simulink library "xblocks_library_ffts_internal"  (Simulink 7.4)
settings: Solver=ode45  StartTime=0.0  StopTime=10.0  RelTol=1e-3
libraries: xbsIndex_r4 x535
(part 1 of 5)
settings Model: Creator=wjm  LastModifiedBy=chenhong

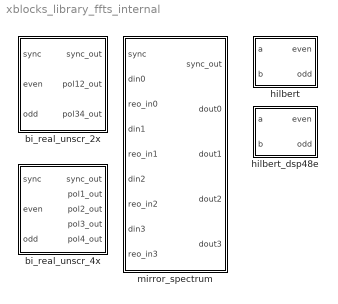
== system xblocks_library_ffts_internal ==
  bi_real_unscr_2x : Subsystem  mask(bi_real_unscr_2x){FFTSize=2, n_bits=18, add_latency=1, conv_latency=1, bram_latency=2, bram_map=off, dsp48_adders=off}
      mask prompts: FFTSize "Size of FFT (2^?):"; n_bits "Sample Bit Width"; add_latency "Add Latency"; conv_latency "Convert Latency"; bram_latency "BRAM Latency"; bram_map "Use BlockRAM for Map"; dsp48_adders "Use DSP48s for adders"
      mask help:
      | FFT internal block.
      |
      | (xBlock version)
      mask init:
      | config.source = str2func('fft_bi_real_unscr_2x_init_xblock');
      | config.toplevel = gcb;
      | config.depend = get_dependlist('fft_bi_real_unscr_2x');
      | set_param(gcb,'LinkStatus','inactive');
      | xBlock( config, {config.toplevel,...
      |     'FFTSize', FFTSize, ...
      |     'n_bits', n_bits, ...
      |     'add_latency', add_latency, ...
      |     'conv_latency', conv_latency, ...
      |     'bram_latency', bram_latency, ...
      |     'bram_map', bram_map, ...
      |     'dsp48_adders', dsp48_adders});
      settings: AttributesFormatString=18_17 r/i
      mask TabNameString: Basic,Basic,Latency,Latency,Latency,Implementation,Implementation
  bi_real_unscr_4x : Subsystem  mask(bi_real_unscr_4x){FFTSize=8, n_bits=18, add_latency=1, conv_latency=1, bram_latency=2, bram_map=off, bram_delays=off, dsp48_adders=on}
      mask prompts: FFTSize "Size of FFT (2^?):"; n_bits "Sample Bit Width"; add_latency "Add Latency"; conv_latency "Convert Latency"; bram_latency "BRAM Latency"; bram_map "Use BlockRAM for Map"; bram_delays "Use BlockRAM for Delays"; dsp48_adders "Use DSP48s for adders"
      mask help:
      | FFT internal block.
      |
      | (xBlock version)
      mask init:
      | config.source = str2func('fft_bi_real_unscr_4x_init_xblock');
      | config.toplevel = gcb;
      | config.depend = get_dependlist('fft_bi_real_unscr_4x');
      | set_param(gcb,'LinkStatus','inactive');
      | xBlock( config, {config.toplevel,...
      |     'FFTSize', FFTSize, ...
      |     'n_bits', n_bits, ...
      |     'add_latency', add_latency, ...
      |     'conv_latency', conv_latency, ...
      |     'bram_latency', bram_latency, ...
      |     'bram_map', bram_map, ...
      |     'bram_delays', bram_delays, ...
      |     'dsp48_adders', dsp48_adders});
      mask TabNameString: Basic,Basic,Latency,Latency,Latency,Implementation,Implementation,Implementation
  hilbert : Subsystem  mask(hilbert (xBlock)){BitWidth=16, add_latency=2, conv_latency=2}
      mask prompts: BitWidth "Bit Wdith"; add_latency "Add Latency"; conv_latency "Convert Latency"
      mask help:
      | FFT internal block.
      |
      | Computes (a+b*)/2 and (a-b*)/2i.
      |
      | If a = w + ix and b = y + iz, then:
      | a+b = (w+y)/2 + i(x-z)/2
      | a-b = (x+z)/2 + i(y-w)/2
      mask init:
      | config.source = str2func('hilbert_init_xblock');
      | config.toplevel = gcb;
      | config.depend = get_dependlist('hilbert');
      | set_param(gcb,'LinkStatus','inactive');
      | xBlock( config, {config.toplevel, ...
      |     BitWidth, add_latency, conv_latency});
  hilbert_dsp48e : Subsystem  mask(sincos_dsp48e (xBlock version)){BitWidth=16, conv_latency=2}
      mask prompts: BitWidth "Bit Wdith"; conv_latency "Convert Latency"
      mask help:
      | FFT internal block.
      |
      | Computes (a+b*)/2 and (a-b*)/2i.
      mask init:
      | config.source = str2func('hilbert_dsp48e_init_xblock');
      | config.toplevel = gcb;
      | config.depend = get_dependlist('hilbert_dsp48e');
      | set_param(gcb,'LinkStatus','inactive');
      | xBlock(config, {config.toplevel, ...
      |     BitWidth, conv_latency});
  mirror_spectrum : Subsystem  mask(mirror_spectrum){FFTSize=8, input_bitwidth=18, bram_latency=2, negate_latency=1, negate_mode=logic}
      mask prompts: FFTSize "Size of FFT (2^?)"; input_bitwidth "Input Bit Width"; bram_latency "BRAM Latency"; negate_latency "Negate Latency"; negate_mode "Negate mode"
      mask help: FFT internal block.
      mask init:
      | config.source = str2func('mirror_spectrum_init_xblock');
      | config.toplevel = gcb;
      | config.depend = get_dependlist('mirror_spectrum');
      | set_param(gcb,'LinkStatus','inactive');
      | xBlock( config, {config.toplevel, ...
      |     FFTSize, input_bitwidth,...
      |     bram_latency, negate_latency, ...
      |     negate_mode});
      settings: AttributesFormatString=18_17 r/i
      mask StyleString: edit,edit,edit,edit,popup(dsp48e|logic)
      mask TabNameString: Basic,Basic,Latency,Latency,Latency

== system xblocks_library_ffts_internal/bi_real_unscr_2x ==
  sync : Inport  OutDataType=sfix(16)  OutScaling=2^0
  even : Inport  Port=2  OutDataType=sfix(16)  OutScaling=2^0
  odd : Inport  Port=3  OutDataType=sfix(16)  OutScaling=2^0
  Constant : xbsIndex_r4/Constant  arith_type=Unsigned  const=0  n_bits=1  bin_pt=0  explicit_period=on  period=1  equ=P=C  opselect=C  inp2=PCIN>>17  opr=+  inp1=P  carry=CIN  dbl_ovrd=off  block_type=constant
      settings: block_version=11.4
  Counter : xbsIndex_r4/Counter  cnt_type=Free Running  cnt_to=Inf  operation=Up  start_count=0  cnt_by_val=1  arith_type=Unsigned  n_bits=1  bin_pt=0  load_pin=off  rst=on  en=off  explicit_period=on  period=1  dbl_ovrd=off  use_behavioral_HDL=off  implementation=Fabric  block_type=counter
      settings: block_version=11.4
  Delay : xbsIndex_r4/Delay  en=off  latency=1  dbl_ovrd=off  reg_retiming=off  block_type=delay
      settings: block_version=11.4
  Mux : xbsIndex_r4/Mux  inputs=2  en=off  latency=0  precision=Full  arith_type="Signed  (2's comp)"  n_bits=8  bin_pt=2  quantization=Truncate  overflow=Wrap  dbl_ovrd=off  block_type=mux
      settings: block_version=11.4
  Relational : xbsIndex_r4/Relational  mode=a=b  en=off  latency=0  dbl_ovrd=off  block_type=relational
  en_even : xbsIndex_r4/Constant  arith_type=Boolean  const=1  n_bits=1  bin_pt=0  explicit_period=on  period=1  equ=P=C  opselect=C  inp2=PCIN>>17  opr=+  inp1=P  carry=CIN  dbl_ovrd=off  block_type=constant
      settings: block_version=11.4
  en_odd : xbsIndex_r4/Constant  arith_type=Boolean  const=1  n_bits=1  bin_pt=0  explicit_period=on  period=1  equ=P=C  opselect=C  inp2=PCIN>>17  opr=+  inp1=P  carry=CIN  dbl_ovrd=off  block_type=constant
      settings: block_version=11.4
  hilbert : Subsystem
      settings: AttributesFormatString=18_17 r/i
  reorder_even : Subsystem
      settings: AttributesFormatString=order=1
  reorder_odd : Subsystem
      settings: AttributesFormatString=order=2
  sync_delay : xbsIndex_r4/Delay  en=off  latency=2  dbl_ovrd=off  reg_retiming=off  block_type=delay
      settings: block_version=11.4
  sync_out : Outport  OutDataType=sfix(16)  OutScaling=2^0
  pol12_out : Outport  Port=2  OutDataType=sfix(16)  OutScaling=2^0
  pol34_out : Outport  Port=3  OutDataType=sfix(16)  OutScaling=2^0
  wires:
  sync/1 -> reorder_odd/1(sync), reorder_even/1(sync)
  reorder_even/1(sync_out) -> sync_delay/1, Counter/1
  reorder_even/3(dout0) -> hilbert/1(a), Mux/3
  reorder_odd/3(dout0) -> Delay/1
  odd/1 -> reorder_odd/3(din0)
  en_odd/1 -> reorder_odd/2(en)
  even/1 -> reorder_even/3(din0)
  en_even/1 -> reorder_even/2(en)
  hilbert/2(odd) -> pol34_out/1
  hilbert/1(even) -> pol12_out/1
  Mux/1 -> hilbert/2(b)
  sync_delay/1 -> sync_out/1
  Relational/1 -> Mux/1
  Constant/1 -> Relational/2
  Counter/1 -> Relational/1
  Delay/1 -> Mux/2

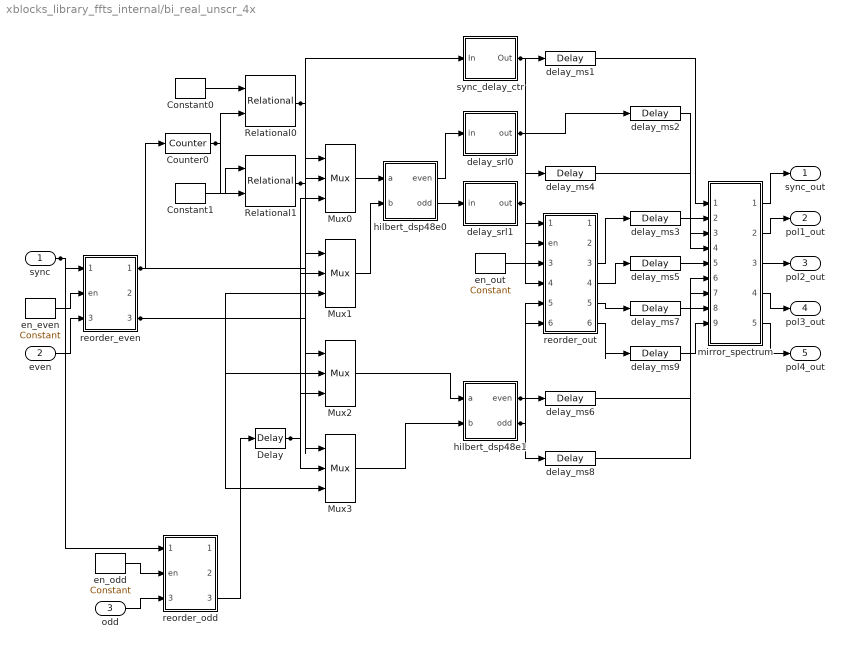
== system xblocks_library_ffts_internal/bi_real_unscr_4x ==
  sync : Inport
  even : Inport  Port=2
  odd : Inport  Port=3
  Constant0 : xbsIndex_r4/Constant  arith_type=Unsigned  const=128  n_bits=8  bin_pt=0  explicit_period=on  period=1  equ=P=C  opselect=C  inp2=PCIN>>17  opr=+  inp1=P  carry=CIN  dbl_ovrd=off  block_type=constant
      settings: block_version=11.4
  Constant1 : xbsIndex_r4/Constant  arith_type=Unsigned  const=0  n_bits=8  bin_pt=0  explicit_period=on  period=1  equ=P=C  opselect=C  inp2=PCIN>>17  opr=+  inp1=P  carry=CIN  dbl_ovrd=off  block_type=constant
      settings: block_version=11.4
  Counter0 : xbsIndex_r4/Counter  cnt_type=Free Running  cnt_to=Inf  operation=Up  start_count=0  cnt_by_val=1  arith_type=Unsigned  n_bits=8  bin_pt=0  load_pin=off  rst=on  en=off  explicit_period=on  period=1  dbl_ovrd=off  use_behavioral_HDL=off  implementation=Fabric  block_type=counter
      settings: block_version=11.4
  Delay : xbsIndex_r4/Delay  en=off  latency=1  dbl_ovrd=off  reg_retiming=off  block_type=delay
      settings: block_version=11.4
  Mux{0..3} (4 alike) : xbsIndex_r4/Mux  inputs=2  en=off  latency=1  precision=Full  arith_type=Unsigned  n_bits=16  bin_pt=14  quantization=Truncate  overflow=Wrap  dbl_ovrd=off  block_type=mux
      settings: block_version=11.4
  Relational0 : xbsIndex_r4/Relational  mode=a=b  en=off  latency=0  dbl_ovrd=off  block_type=relational
  Relational1 : xbsIndex_r4/Relational  mode=a=b  en=off  latency=0  dbl_ovrd=off  block_type=relational
  delay_ms{1..9} (9 alike) : xbsIndex_r4/Delay  en=off  latency=1  dbl_ovrd=off  reg_retiming=off  block_type=delay
      settings: block_version=11.4
  delay_srl0 : Subsystem
  delay_srl1 : Subsystem
  en_even : xbsIndex_r4/Constant  arith_type=Boolean  const=1  n_bits=1  bin_pt=0  explicit_period=on  period=1  equ=P=C  opselect=C  inp2=PCIN>>17  opr=+  inp1=P  carry=CIN  dbl_ovrd=off  block_type=constant
      settings: block_version=11.4
  en_odd : xbsIndex_r4/Constant  arith_type=Boolean  const=1  n_bits=1  bin_pt=0  explicit_period=on  period=1  equ=P=C  opselect=C  inp2=PCIN>>17  opr=+  inp1=P  carry=CIN  dbl_ovrd=off  block_type=constant
      settings: block_version=11.4
  en_out : xbsIndex_r4/Constant  arith_type=Boolean  const=1  n_bits=1  bin_pt=0  explicit_period=on  period=1  equ=P=C  opselect=C  inp2=PCIN>>17  opr=+  inp1=P  carry=CIN  dbl_ovrd=off  block_type=constant
      settings: block_version=11.4
  hilbert_dsp48e0 : Subsystem
  hilbert_dsp48e1 : Subsystem
  mirror_spectrum : Subsystem
  reorder_even : Subsystem
      settings: AttributesFormatString=order=2
  reorder_odd : Subsystem
      settings: AttributesFormatString=order=2
  reorder_out : Subsystem
      settings: AttributesFormatString=order=2
  sync_delay_ctr : Subsystem
  sync_out : Outport
  pol1_out : Outport  Port=2
  pol2_out : Outport  Port=3
  pol3_out : Outport  Port=4
  pol4_out : Outport  Port=5
  wires:
  sync/1 -> reorder_odd/1(sync), reorder_even/1(sync)
  reorder_even/1(sync_out) -> sync_delay_ctr/1(In), Counter0/1
  Counter0/1 -> Relational1/2, Relational0/2
  Relational0/1 -> Mux3/1, Mux0/1
  reorder_even/3(dout0) -> Mux3/3, Mux2/2, Mux1/3, Mux0/2
  Delay/1 -> Mux3/2, Mux2/3, Mux1/2, Mux0/3
  Relational1/1 -> Mux2/1, Mux1/1
  sync_delay_ctr/1(Out) -> delay_ms1/1, reorder_out/1(sync)
  delay_srl0/1(out) -> delay_ms2/1, reorder_out/3(din0)
  delay_srl1/1(out) -> delay_ms4/1, reorder_out/4(din1)
  hilbert_dsp48e1/1(even) -> delay_ms6/1, reorder_out/5(din2)
  hilbert_dsp48e1/2(odd) -> delay_ms8/1, reorder_out/6(din3)
  mirror_spectrum/5(dout3) -> pol4_out/1
  mirror_spectrum/4(dout2) -> pol3_out/1
  mirror_spectrum/3(dout1) -> pol2_out/1
  mirror_spectrum/2(dout0) -> pol1_out/1
  mirror_spectrum/1(sync_out) -> sync_out/1
  delay_ms9/1 -> mirror_spectrum/9(reo_in3)
  delay_ms8/1 -> mirror_spectrum/8(din3)
  delay_ms7/1 -> mirror_spectrum/7(reo_in2)
  delay_ms6/1 -> mirror_spectrum/6(din2)
  delay_ms5/1 -> mirror_spectrum/5(reo_in1)
  delay_ms4/1 -> mirror_spectrum/4(din1)
  delay_ms3/1 -> mirror_spectrum/3(reo_in0)
  delay_ms2/1 -> mirror_spectrum/2(din0)
  delay_ms1/1 -> mirror_spectrum/1(sync)
  reorder_out/6(dout3) -> delay_ms9/1
  reorder_out/5(dout2) -> delay_ms7/1
  reorder_out/4(dout1) -> delay_ms5/1
  reorder_out/3(dout0) -> delay_ms3/1
  en_out/1 -> reorder_out/2(en)
  hilbert_dsp48e0/2(odd) -> delay_srl1/1(in)
  hilbert_dsp48e0/1(even) -> delay_srl0/1(in)
  Mux3/1 -> hilbert_dsp48e1/2(b)
  Mux2/1 -> hilbert_dsp48e1/1(a)
  Mux1/1 -> hilbert_dsp48e0/2(b)
  Mux0/1 -> hilbert_dsp48e0/1(a)
  reorder_odd/3(dout0) -> Delay/1
  Constant1/1 -> Relational1/1
  Constant0/1 -> Relational0/1
  odd/1 -> reorder_odd/3(din0)
  en_odd/1 -> reorder_odd/2(en)
  even/1 -> reorder_even/3(din0)
  en_even/1 -> reorder_even/2(en)

== system xblocks_library_ffts_internal/hilbert ==
  a : Inport  OutDataType=sfix(16)  OutScaling=2^0
  b : Inport  Port=2  OutDataType=sfix(16)  OutScaling=2^0
  AddSub : xbsIndex_r4/AddSub  mode=Addition  use_carryin=off  use_carryout=off  en=off  latency=2  precision=Full  arith_type=Unsigned  n_bits=8  bin_pt=2  quantization=Truncate  overflow=Wrap  dbl_ovrd=off  use_behavioral_HDL=on  hw_selection=Fabric  pipelined=off  use_rpm=on  block_type=addsub
  AddSub1 : xbsIndex_r4/AddSub  mode=Subtraction  use_carryin=off  use_carryout=off  en=off  latency=2  precision=Full  arith_type=Unsigned  n_bits=8  bin_pt=2  quantization=Truncate  overflow=Wrap  dbl_ovrd=off  use_behavioral_HDL=on  hw_selection=Fabric  pipelined=off  use_rpm=on  block_type=addsub
  AddSub2 : xbsIndex_r4/AddSub  mode=Subtraction  use_carryin=off  use_carryout=off  en=off  latency=2  precision=Full  arith_type=Unsigned  n_bits=8  bin_pt=2  quantization=Truncate  overflow=Wrap  dbl_ovrd=off  use_behavioral_HDL=on  hw_selection=Fabric  pipelined=off  use_rpm=on  block_type=addsub
  AddSub3 : xbsIndex_r4/AddSub  mode=Addition  use_carryin=off  use_carryout=off  en=off  latency=2  precision=Full  arith_type=Unsigned  n_bits=8  bin_pt=2  quantization=Truncate  overflow=Wrap  dbl_ovrd=off  use_behavioral_HDL=on  hw_selection=Fabric  pipelined=off  use_rpm=on  block_type=addsub
  Convert{,1..3} (4 alike) : xbsIndex_r4/Convert  arith_type="Signed  (2's comp)"  n_bits=16  bin_pt=15  quantization="Round  (unbiased: Even Values)"  overflow=Wrap  latency=2  dbl_ovrd=off  pipeline=off  block_type=convert
      settings: block_version=11.4
  Scale{,1..3} (4 alike) : xbsIndex_r4/Scale  scale_factor=-1  dbl_ovrd=off  block_type=scale
  c_to_ri : Subsystem
      settings: AttributesFormatString=16_15 r/i
  c_to_ri1 : Subsystem
      settings: AttributesFormatString=16_15 r/i
  ri_to_c : Subsystem
  ri_to_c1 : Subsystem
  even : Outport  OutDataType=sfix(16)  OutScaling=2^0
  odd : Outport  Port=2  OutDataType=sfix(16)  OutScaling=2^0
  wires:
  c_to_ri/1(re) -> AddSub1/2, AddSub/1
  c_to_ri/2(im) -> AddSub3/1, AddSub2/1
  c_to_ri1/1(re) -> AddSub1/1, AddSub/2
  c_to_ri1/2(im) -> AddSub3/2, AddSub2/2
  ri_to_c1/1(c) -> odd/1
  Convert1/1 -> ri_to_c1/2(im)
  Convert3/1 -> ri_to_c1/1(re)
  ri_to_c/1(c) -> even/1
  Convert2/1 -> ri_to_c/2(im)
  Convert/1 -> ri_to_c/1(re)
  b/1 -> c_to_ri1/1(c)
  a/1 -> c_to_ri/1(c)
  Scale3/1 -> Convert3/1
  AddSub3/1 -> Scale3/1
  Scale2/1 -> Convert2/1
  AddSub2/1 -> Scale2/1
  Scale1/1 -> Convert1/1
  AddSub1/1 -> Scale1/1
  Scale/1 -> Convert/1
  AddSub/1 -> Scale/1

== system xblocks_library_ffts_internal/hilbert_dsp48e ==
  a : Inport
  b : Inport  Port=2
  Convert{0..3} (4 alike) : xbsIndex_r4/Convert  arith_type="Signed  (2's comp)"  n_bits=16  bin_pt=15  quantization="Round  (unbiased: Even Values)"  overflow=Wrap  latency=2  dbl_ovrd=off  pipeline=on  block_type=convert
      settings: block_version=11.4
  Scale{0..3} (4 alike) : xbsIndex_r4/Scale  scale_factor=-1  dbl_ovrd=off  block_type=scale
  c_to_ri0 : Subsystem
      settings: AttributesFormatString=16_15 r/i
  c_to_ri1 : Subsystem
      settings: AttributesFormatString=16_15 r/i
  cadd : Subsystem
      settings: AttributesFormatString=|
      | 16_15 + 16_15 ==> 17_15
      | Mode=Addition
      | Latency=2
  csub : Subsystem
      settings: AttributesFormatString=|
      | 16_15 + 16_15 ==> 17_15
      | Mode=Subtraction
      | Latency=2
  ri_to_c0 : Subsystem
  ri_to_c1 : Subsystem
  even : Outport
  odd : Outport  Port=2
  wires:
  c_to_ri0/1(re) -> csub/4(b_im), cadd/1(a_re)
  c_to_ri0/2(im) -> csub/1(a_re), cadd/2(a_im)
  c_to_ri1/1(re) -> csub/2(a_im), cadd/3(b_re)
  c_to_ri1/2(im) -> csub/3(b_re), cadd/4(b_im)
  ri_to_c1/1(c) -> odd/1
  Convert3/1 -> ri_to_c1/2(im)
  Convert1/1 -> ri_to_c1/1(re)
  ri_to_c0/1(c) -> even/1
  Convert2/1 -> ri_to_c0/2(im)
  Convert0/1 -> ri_to_c0/1(re)
  csub/2(c_im) -> Scale3/1
  csub/1(c_re) -> Scale2/1
  cadd/2(c_im) -> Scale1/1
  cadd/1(c_re) -> Scale0/1
  b/1 -> c_to_ri1/1(c)
  a/1 -> c_to_ri0/1(c)
  Scale3/1 -> Convert3/1
  Scale2/1 -> Convert2/1
  Scale1/1 -> Convert1/1
  Scale0/1 -> Convert0/1

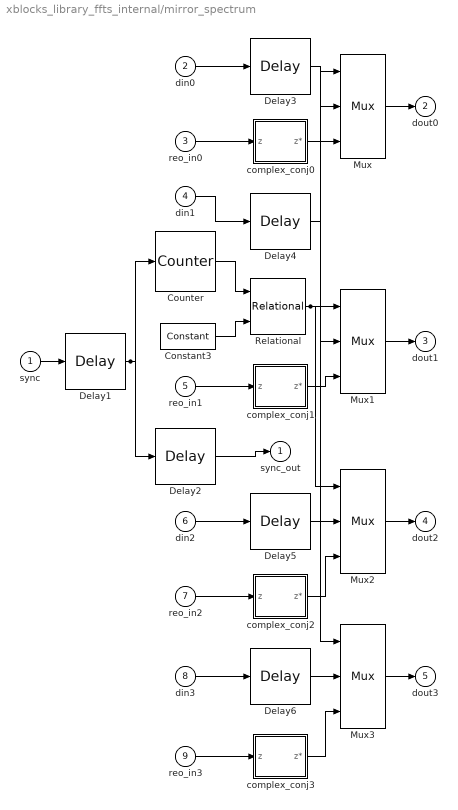
== system xblocks_library_ffts_internal/mirror_spectrum ==
  sync : Inport
  din0 : Inport  Port=2
  reo_in0 : Inport  Port=3
  din1 : Inport  Port=4
  reo_in1 : Inport  Port=5
  din2 : Inport  Port=6
  reo_in2 : Inport  Port=7
  din3 : Inport  Port=8
  reo_in3 : Inport  Port=9
  Constant3 : xbsIndex_r4/Constant  arith_type=Unsigned  const=128  n_bits=8  bin_pt=0  explicit_period=on  period=1  equ=P=C  opselect=C  inp2=PCIN>>17  opr=+  inp1=P  carry=CIN  dbl_ovrd=off  block_type=constant
      settings: block_version=11.4
  Counter : xbsIndex_r4/Counter  cnt_type=Free Running  cnt_to=Inf  operation=Up  start_count=0  cnt_by_val=1  arith_type=Unsigned  n_bits=8  bin_pt=0  load_pin=off  rst=on  en=off  explicit_period=off  period=1  dbl_ovrd=off  use_behavioral_HDL=off  implementation=Fabric  use_rpm=on  block_type=counter
      settings: block_version=11.4
  Delay1 : xbsIndex_r4/Delay  en=off  latency=2  dbl_ovrd=off  reg_retiming=off  block_type=delay
      settings: block_version=11.4
  Delay2 : xbsIndex_r4/Delay  en=off  latency=2  dbl_ovrd=off  reg_retiming=off  block_type=delay
      settings: block_version=11.4
  Delay{3..6} (4 alike) : xbsIndex_r4/Delay  en=off  latency=3  dbl_ovrd=off  reg_retiming=off  block_type=delay
      settings: block_version=11.4
  Mux{,1..3} (4 alike) : xbsIndex_r4/Mux  inputs=2  en=off  latency=1  precision=Full  arith_type="Signed  (2's comp)"  n_bits=8  bin_pt=2  quantization=Truncate  overflow=Wrap  dbl_ovrd=off  block_type=mux
      settings: block_version=11.4
  Relational : xbsIndex_r4/Relational  mode=a>b  en=off  latency=1  dbl_ovrd=off  block_type=relational
  complex_conj0 : Subsystem
      settings: AttributesFormatString=18_17 r/i
  complex_conj1 : Subsystem
      settings: AttributesFormatString=18_17 r/i
  complex_conj2 : Subsystem
      settings: AttributesFormatString=18_17 r/i
  complex_conj3 : Subsystem
      settings: AttributesFormatString=18_17 r/i
  sync_out : Outport
  dout0 : Outport  Port=2
  dout1 : Outport  Port=3
  dout2 : Outport  Port=4
  dout3 : Outport  Port=5
  wires:
  Delay1/1 -> Delay2/1, Counter/1
  Relational/1 -> Mux3/1, Mux2/1, Mux1/1, Mux/1
  complex_conj3/1(z*) -> Mux3/3
  reo_in3/1 -> complex_conj3/1(z)
  complex_conj2/1(z*) -> Mux2/3
  reo_in2/1 -> complex_conj2/1(z)
  complex_conj1/1(z*) -> Mux1/3
  reo_in1/1 -> complex_conj1/1(z)
  complex_conj0/1(z*) -> Mux/3
  reo_in0/1 -> complex_conj0/1(z)
  Constant3/1 -> Relational/2
  Counter/1 -> Relational/1
  Mux3/1 -> dout3/1
  Delay6/1 -> Mux3/2
  Mux2/1 -> dout2/1
  Delay5/1 -> Mux2/2
  Mux1/1 -> dout1/1
  Delay4/1 -> Mux1/2
  Mux/1 -> dout0/1
  Delay3/1 -> Mux/2
  din3/1 -> Delay6/1
  din2/1 -> Delay5/1
  din1/1 -> Delay4/1
  din0/1 -> Delay3/1
  Delay2/1 -> sync_out/1
  sync/1 -> Delay1/1

== system xblocks_library_ffts_internal/bi_real_unscr_2x/hilbert ==
  a : Inport
  b : Inport  Port=2
  AddSub : xbsIndex_r4/AddSub  mode=Addition  use_carryin=off  use_carryout=off  en=off  latency=1  precision=Full  arith_type=Unsigned  n_bits=8  bin_pt=2  quantization=Truncate  overflow=Wrap  dbl_ovrd=off  use_behavioral_HDL=on  hw_selection=Fabric  pipelined=off  use_rpm=on  block_type=addsub
  AddSub1 : xbsIndex_r4/AddSub  mode=Subtraction  use_carryin=off  use_carryout=off  en=off  latency=1  precision=Full  arith_type=Unsigned  n_bits=8  bin_pt=2  quantization=Truncate  overflow=Wrap  dbl_ovrd=off  use_behavioral_HDL=on  hw_selection=Fabric  pipelined=off  use_rpm=on  block_type=addsub
  AddSub2 : xbsIndex_r4/AddSub  mode=Subtraction  use_carryin=off  use_carryout=off  en=off  latency=1  precision=Full  arith_type=Unsigned  n_bits=8  bin_pt=2  quantization=Truncate  overflow=Wrap  dbl_ovrd=off  use_behavioral_HDL=on  hw_selection=Fabric  pipelined=off  use_rpm=on  block_type=addsub
  AddSub3 : xbsIndex_r4/AddSub  mode=Addition  use_carryin=off  use_carryout=off  en=off  latency=1  precision=Full  arith_type=Unsigned  n_bits=8  bin_pt=2  quantization=Truncate  overflow=Wrap  dbl_ovrd=off  use_behavioral_HDL=on  hw_selection=Fabric  pipelined=off  use_rpm=on  block_type=addsub
  Convert{,1..3} (4 alike) : xbsIndex_r4/Convert  arith_type="Signed  (2's comp)"  n_bits=18  bin_pt=17  quantization="Round  (unbiased: Even Values)"  overflow=Wrap  latency=1  dbl_ovrd=off  pipeline=off  block_type=convert
      settings: block_version=11.4
  Scale{,1..3} (4 alike) : xbsIndex_r4/Scale  scale_factor=-1  dbl_ovrd=off  block_type=scale
  c_to_ri : Subsystem
  c_to_ri1 : Subsystem
  ri_to_c : Subsystem
  ri_to_c1 : Subsystem
  even : Outport
  odd : Outport  Port=2
  wires:
  c_to_ri/1(re) -> AddSub1/2, AddSub/1
  c_to_ri/2(im) -> AddSub3/1, AddSub2/1
  c_to_ri1/1(re) -> AddSub1/1, AddSub/2
  c_to_ri1/2(im) -> AddSub3/2, AddSub2/2
  ri_to_c1/1(c) -> odd/1
  Convert1/1 -> ri_to_c1/2(im)
  Convert3/1 -> ri_to_c1/1(re)
  ri_to_c/1(c) -> even/1
  Convert2/1 -> ri_to_c/2(im)
  Convert/1 -> ri_to_c/1(re)
  b/1 -> c_to_ri1/1(c)
  a/1 -> c_to_ri/1(c)
  Scale3/1 -> Convert3/1
  AddSub3/1 -> Scale3/1
  Scale2/1 -> Convert2/1
  AddSub2/1 -> Scale2/1
  Scale1/1 -> Convert1/1
  AddSub1/1 -> Scale1/1
  Scale/1 -> Convert/1
  AddSub/1 -> Scale/1

== system xblocks_library_ffts_internal/bi_real_unscr_2x/reorder_even ==
  sync : Inport
  en : Inport  Port=2
  din0 : Inport  Port=3
  delay_din1 : xbsIndex_r4/Delay  en=off  latency=1  dbl_ovrd=off  reg_retiming=off  block_type=delay
      settings: block_version=11.4
  delay_din_bram0 : Subsystem
  delay_valid : xbsIndex_r4/Delay  en=off  latency=3  dbl_ovrd=off  reg_retiming=off  block_type=delay
      settings: block_version=11.4
  delay_we : xbsIndex_r4/Delay  en=off  latency=0  dbl_ovrd=off  reg_retiming=off  block_type=delay
      settings: block_version=11.4
  post_sync_delay : xbsIndex_r4/Delay  en=off  latency=3  dbl_ovrd=off  reg_retiming=off  block_type=delay
      settings: block_version=11.4
  pre_sync_delay : xbsIndex_r4/Delay  en=off  latency=0  dbl_ovrd=off  reg_retiming=off  block_type=delay
      settings: block_version=11.4
  sync_delay_en : Subsystem
  sync_out : Outport
  valid : Outport  Port=2
  dout0 : Outport  Port=3
  wires:
  en/1 -> delay_we/1, sync_delay_en/2(en)
  delay_we/1 -> delay_din_bram0/2(en), delay_valid/1
  delay_din_bram0/1(dout) -> dout0/1
  delay_din1/1 -> delay_din_bram0/1(din)
  din0/1 -> delay_din1/1
  delay_valid/1 -> valid/1
  post_sync_delay/1 -> sync_out/1
  sync_delay_en/1(Out) -> post_sync_delay/1
  pre_sync_delay/1 -> sync_delay_en/1(In)
  sync/1 -> pre_sync_delay/1

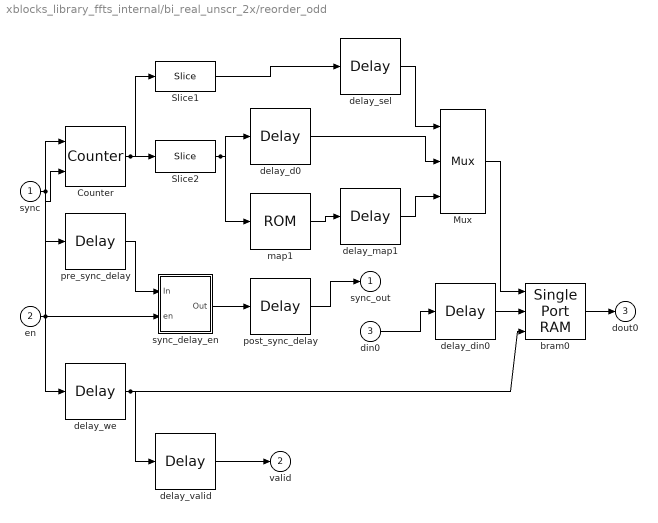
== system xblocks_library_ffts_internal/bi_real_unscr_2x/reorder_odd ==
  sync : Inport
  en : Inport  Port=2
  din0 : Inport  Port=3
  Counter : xbsIndex_r4/Counter  cnt_type=Count Limited  cnt_to=3  operation=Up  start_count=0  cnt_by_val=1  arith_type=Unsigned  n_bits=2  bin_pt=0  load_pin=off  rst=on  en=on  explicit_period=on  period=1  dbl_ovrd=off  use_behavioral_HDL=off  implementation=Fabric  block_type=counter
      settings: block_version=11.4
  Mux : xbsIndex_r4/Mux  inputs=2  en=off  latency=1  precision=Full  arith_type=Unsigned  n_bits=16  bin_pt=14  quantization=Truncate  overflow=Wrap  dbl_ovrd=off  block_type=mux
      settings: block_version=11.4
  Slice1 : xbsIndex_r4/Slice  nbits=1  boolean_output=off  mode=Upper Bit Location + Width  bit1=0  base1=MSB of Input  bit0=0  base0=LSB of Input  dbl_ovrd=off  block_type=slice
  Slice2 : xbsIndex_r4/Slice  nbits=1  boolean_output=off  mode=Lower Bit Location + Width  bit1=0  base1=MSB of Input  bit0=0  base0=LSB of Input  dbl_ovrd=off  block_type=slice
  bram0 : xbsIndex_r4/Single Port RAM  depth=2  initVector=sin(pi*(0:15)/16)  distributed_mem=Block RAM  write_mode=Read Before Write  rst=off  init_reg=0  en=off  latency=2  dbl_ovrd=off  optimize=Area  use_rpm=on  block_type=spram
  delay_d0 : xbsIndex_r4/Delay  en=off  latency=1  dbl_ovrd=off  reg_retiming=off  block_type=delay
      settings: block_version=11.4
  delay_din0 : xbsIndex_r4/Delay  en=off  latency=2  dbl_ovrd=off  reg_retiming=off  block_type=delay
      settings: block_version=11.4
  delay_map1 : xbsIndex_r4/Delay  en=off  latency=0  dbl_ovrd=off  reg_retiming=off  block_type=delay
      settings: block_version=11.4
  delay_sel : xbsIndex_r4/Delay  en=off  latency=1  dbl_ovrd=off  reg_retiming=off  block_type=delay
      settings: block_version=11.4
  delay_valid : xbsIndex_r4/Delay  en=off  latency=3  dbl_ovrd=off  reg_retiming=off  block_type=delay
      settings: block_version=11.4
  delay_we : xbsIndex_r4/Delay  en=off  latency=1  dbl_ovrd=off  reg_retiming=off  block_type=delay
      settings: block_version=11.4
  map1 : xbsIndex_r4/ROM  depth=2  initVector=[1 0]  distributed_mem=Distributed memory  rst=off  init_reg=0  en=off  latency=1  arith_type=Unsigned  n_bits=1  bin_pt=0  dbl_ovrd=off  optimize=Area  use_rpm=on  block_type=sprom
      settings: block_version=11.4
  post_sync_delay : xbsIndex_r4/Delay  en=off  latency=3  dbl_ovrd=off  reg_retiming=off  block_type=delay
      settings: block_version=11.4
  pre_sync_delay : xbsIndex_r4/Delay  en=off  latency=1  dbl_ovrd=off  reg_retiming=off  block_type=delay
      settings: block_version=11.4
  sync_delay_en : Subsystem
  sync_out : Outport
  valid : Outport  Port=2
  dout0 : Outport  Port=3
  wires:
  sync/1 -> Counter/1, pre_sync_delay/1
  en/1 -> Counter/2, delay_we/1, sync_delay_en/2(en)
  delay_we/1 -> bram0/3, delay_valid/1
  Counter/1 -> Slice2/1, Slice1/1
  Slice2/1 -> map1/1, delay_d0/1
  delay_map1/1 -> Mux/3
  map1/1 -> delay_map1/1
  bram0/1 -> dout0/1
  delay_din0/1 -> bram0/2
  Mux/1 -> bram0/1
  din0/1 -> delay_din0/1
  delay_d0/1 -> Mux/2
  delay_sel/1 -> Mux/1
  Slice1/1 -> delay_sel/1
  delay_valid/1 -> valid/1
  post_sync_delay/1 -> sync_out/1
  sync_delay_en/1(Out) -> post_sync_delay/1
  pre_sync_delay/1 -> sync_delay_en/1(In)

== system xblocks_library_ffts_internal/bi_real_unscr_4x/delay_srl0 ==
  in : Inport
  delay_ff : xbsIndex_r4/Delay  en=off  latency=1  dbl_ovrd=off  reg_retiming=off  block_type=delay
      settings: block_version=11.4
  delay_srl : xbsIndex_r4/Delay  en=off  latency=127  dbl_ovrd=off  reg_retiming=off  block_type=delay
      settings: block_version=11.4
  out : Outport
  wires:
  delay_srl/1 -> out/1
  delay_ff/1 -> delay_srl/1
  in/1 -> delay_ff/1

== system xblocks_library_ffts_internal/bi_real_unscr_4x/delay_srl1 ==
  in : Inport
  delay_ff : xbsIndex_r4/Delay  en=off  latency=1  dbl_ovrd=off  reg_retiming=off  block_type=delay
      settings: block_version=11.4
  delay_srl : xbsIndex_r4/Delay  en=off  latency=127  dbl_ovrd=off  reg_retiming=off  block_type=delay
      settings: block_version=11.4
  out : Outport
  wires:
  delay_srl/1 -> out/1
  delay_ff/1 -> delay_srl/1
  in/1 -> delay_ff/1

== system xblocks_library_ffts_internal/bi_real_unscr_4x/hilbert_dsp48e0 ==
  a : Inport
  b : Inport  Port=2
  Convert{0..3} (4 alike) : xbsIndex_r4/Convert  arith_type="Signed  (2's comp)"  n_bits=18  bin_pt=17  quantization="Round  (unbiased: Even Values)"  overflow=Wrap  latency=1  dbl_ovrd=off  pipeline=on  block_type=convert
      settings: block_version=11.4
  Scale{0..3} (4 alike) : xbsIndex_r4/Scale  scale_factor=-1  dbl_ovrd=off  block_type=scale
  c_to_ri0 : Subsystem
  c_to_ri1 : Subsystem
  cadd : Subsystem
      settings: AttributesFormatString=|
      | 18_17 + 18_17 ==> 19_17
      | Mode=Addition
      | Latency=2
  csub : Subsystem
      settings: AttributesFormatString=|
      | 18_17 + 18_17 ==> 19_17
      | Mode=Subtraction
      | Latency=2
  ri_to_c0 : Subsystem
  ri_to_c1 : Subsystem
  even : Outport
  odd : Outport  Port=2
  wires:
  c_to_ri0/1(re) -> csub/4(b_im), cadd/1(a_re)
  c_to_ri0/2(im) -> csub/1(a_re), cadd/2(a_im)
  c_to_ri1/1(re) -> csub/2(a_im), cadd/3(b_re)
  c_to_ri1/2(im) -> csub/3(b_re), cadd/4(b_im)
  ri_to_c1/1(c) -> odd/1
  Convert3/1 -> ri_to_c1/2(im)
  Convert1/1 -> ri_to_c1/1(re)
  ri_to_c0/1(c) -> even/1
  Convert2/1 -> ri_to_c0/2(im)
  Convert0/1 -> ri_to_c0/1(re)
  csub/2(c_im) -> Scale3/1
  csub/1(c_re) -> Scale2/1
  cadd/2(c_im) -> Scale1/1
  cadd/1(c_re) -> Scale0/1
  b/1 -> c_to_ri1/1(c)
  a/1 -> c_to_ri0/1(c)
  Scale3/1 -> Convert3/1
  Scale2/1 -> Convert2/1
  Scale1/1 -> Convert1/1
  Scale0/1 -> Convert0/1

== system xblocks_library_ffts_internal/bi_real_unscr_4x/hilbert_dsp48e1 ==
  a : Inport
  b : Inport  Port=2
  Convert{0..3} (4 alike) : xbsIndex_r4/Convert  arith_type="Signed  (2's comp)"  n_bits=18  bin_pt=17  quantization="Round  (unbiased: Even Values)"  overflow=Wrap  latency=1  dbl_ovrd=off  pipeline=on  block_type=convert
      settings: block_version=11.4
  Scale{0..3} (4 alike) : xbsIndex_r4/Scale  scale_factor=-1  dbl_ovrd=off  block_type=scale
  c_to_ri0 : Subsystem
  c_to_ri1 : Subsystem
  cadd : Subsystem
      settings: AttributesFormatString=|
      | 18_17 + 18_17 ==> 19_17
      | Mode=Addition
      | Latency=2
  csub : Subsystem
      settings: AttributesFormatString=|
      | 18_17 + 18_17 ==> 19_17
      | Mode=Subtraction
      | Latency=2
  ri_to_c0 : Subsystem
  ri_to_c1 : Subsystem
  even : Outport
  odd : Outport  Port=2
  wires:
  c_to_ri0/1(re) -> csub/4(b_im), cadd/1(a_re)
  c_to_ri0/2(im) -> csub/1(a_re), cadd/2(a_im)
  c_to_ri1/1(re) -> csub/2(a_im), cadd/3(b_re)
  c_to_ri1/2(im) -> csub/3(b_re), cadd/4(b_im)
  ri_to_c1/1(c) -> odd/1
  Convert3/1 -> ri_to_c1/2(im)
  Convert1/1 -> ri_to_c1/1(re)
  ri_to_c0/1(c) -> even/1
  Convert2/1 -> ri_to_c0/2(im)
  Convert0/1 -> ri_to_c0/1(re)
  csub/2(c_im) -> Scale3/1
  csub/1(c_re) -> Scale2/1
  cadd/2(c_im) -> Scale1/1
  cadd/1(c_re) -> Scale0/1
  b/1 -> c_to_ri1/1(c)
  a/1 -> c_to_ri0/1(c)
  Scale3/1 -> Convert3/1
  Scale2/1 -> Convert2/1
  Scale1/1 -> Convert1/1
  Scale0/1 -> Convert0/1

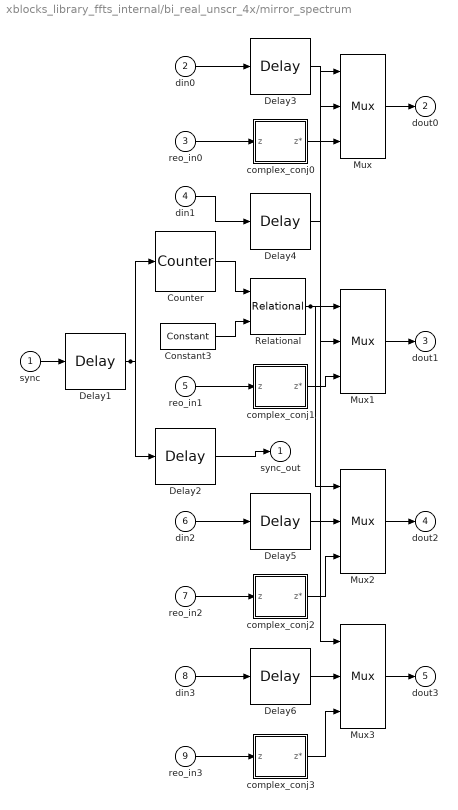
== system xblocks_library_ffts_internal/bi_real_unscr_4x/mirror_spectrum ==
  sync : Inport
  din0 : Inport  Port=2
  reo_in0 : Inport  Port=3
  din1 : Inport  Port=4
  reo_in1 : Inport  Port=5
  din2 : Inport  Port=6
  reo_in2 : Inport  Port=7
  din3 : Inport  Port=8
  reo_in3 : Inport  Port=9
  Constant3 : xbsIndex_r4/Constant  arith_type=Unsigned  const=128  n_bits=8  bin_pt=0  explicit_period=on  period=1  equ=P=C  opselect=C  inp2=PCIN>>17  opr=+  inp1=P  carry=CIN  dbl_ovrd=off  block_type=constant
      settings: block_version=11.4
  Counter : xbsIndex_r4/Counter  cnt_type=Free Running  cnt_to=Inf  operation=Up  start_count=0  cnt_by_val=1  arith_type=Unsigned  n_bits=8  bin_pt=0  load_pin=off  rst=on  en=off  explicit_period=off  period=1  dbl_ovrd=off  use_behavioral_HDL=off  implementation=Fabric  use_rpm=on  block_type=counter
      settings: block_version=11.4
  Delay1 : xbsIndex_r4/Delay  en=off  latency=2  dbl_ovrd=off  reg_retiming=off  block_type=delay
      settings: block_version=11.4
  Delay2 : xbsIndex_r4/Delay  en=off  latency=2  dbl_ovrd=off  reg_retiming=off  block_type=delay
      settings: block_version=11.4
  Delay{3..6} (4 alike) : xbsIndex_r4/Delay  en=off  latency=3  dbl_ovrd=off  reg_retiming=off  block_type=delay
      settings: block_version=11.4
  Mux{,1..3} (4 alike) : xbsIndex_r4/Mux  inputs=2  en=off  latency=1  precision=Full  arith_type="Signed  (2's comp)"  n_bits=8  bin_pt=2  quantization=Truncate  overflow=Wrap  dbl_ovrd=off  block_type=mux
      settings: block_version=11.4
  Relational : xbsIndex_r4/Relational  mode=a>b  en=off  latency=1  dbl_ovrd=off  block_type=relational
  complex_conj0 : Subsystem
  complex_conj1 : Subsystem
  complex_conj2 : Subsystem
  complex_conj3 : Subsystem
  sync_out : Outport
  dout0 : Outport  Port=2
  dout1 : Outport  Port=3
  dout2 : Outport  Port=4
  dout3 : Outport  Port=5
  wires:
  Delay1/1 -> Delay2/1, Counter/1
  Relational/1 -> Mux3/1, Mux2/1, Mux1/1, Mux/1
  complex_conj3/1(z*) -> Mux3/3
  reo_in3/1 -> complex_conj3/1(z)
  complex_conj2/1(z*) -> Mux2/3
  reo_in2/1 -> complex_conj2/1(z)
  complex_conj1/1(z*) -> Mux1/3
  reo_in1/1 -> complex_conj1/1(z)
  complex_conj0/1(z*) -> Mux/3
  reo_in0/1 -> complex_conj0/1(z)
  Constant3/1 -> Relational/2
  Counter/1 -> Relational/1
  Mux3/1 -> dout3/1
  Delay6/1 -> Mux3/2
  Mux2/1 -> dout2/1
  Delay5/1 -> Mux2/2
  Mux1/1 -> dout1/1
  Delay4/1 -> Mux1/2
  Mux/1 -> dout0/1
  Delay3/1 -> Mux/2
  din3/1 -> Delay6/1
  din2/1 -> Delay5/1
  din1/1 -> Delay4/1
  din0/1 -> Delay3/1
  Delay2/1 -> sync_out/1
  sync/1 -> Delay1/1

== system xblocks_library_ffts_internal/bi_real_unscr_4x/reorder_even ==
  sync : Inport
  en : Inport  Port=2
  din0 : Inport  Port=3
  Counter : xbsIndex_r4/Counter  cnt_type=Count Limited  cnt_to=255  operation=Up  start_count=0  cnt_by_val=1  arith_type=Unsigned  n_bits=8  bin_pt=0  load_pin=off  rst=on  en=on  explicit_period=on  period=1  dbl_ovrd=off  use_behavioral_HDL=off  implementation=Fabric  block_type=counter
      settings: block_version=11.4
  Mux : xbsIndex_r4/Mux  inputs=2  en=off  latency=1  precision=Full  arith_type=Unsigned  n_bits=16  bin_pt=14  quantization=Truncate  overflow=Wrap  dbl_ovrd=off  block_type=mux
      settings: block_version=11.4
  Slice1 : xbsIndex_r4/Slice  nbits=1  boolean_output=off  mode=Upper Bit Location + Width  bit1=0  base1=MSB of Input  bit0=0  base0=LSB of Input  dbl_ovrd=off  block_type=slice
  Slice2 : xbsIndex_r4/Slice  nbits=7  boolean_output=off  mode=Lower Bit Location + Width  bit1=0  base1=MSB of Input  bit0=0  base0=LSB of Input  dbl_ovrd=off  block_type=slice
  bram0 : xbsIndex_r4/Single Port RAM  depth=128  initVector=sin(pi*(0:15)/16)  distributed_mem=Block RAM  write_mode=Read Before Write  rst=off  init_reg=0  en=off  latency=2  dbl_ovrd=off  optimize=Area  use_rpm=on  block_type=spram
  delay_d0 : xbsIndex_r4/Delay  en=off  latency=0  dbl_ovrd=off  reg_retiming=off  block_type=delay
      settings: block_version=11.4
  delay_din0 : xbsIndex_r4/Delay  en=off  latency=1  dbl_ovrd=off  reg_retiming=off  block_type=delay
      settings: block_version=11.4
  delay_map1 : xbsIndex_r4/Delay  en=off  latency=0  dbl_ovrd=off  reg_retiming=off  block_type=delay
      settings: block_version=11.4
  delay_sel : xbsIndex_r4/Delay  en=off  latency=0  dbl_ovrd=off  reg_retiming=off  block_type=delay
      settings: block_version=11.4
  delay_valid : xbsIndex_r4/Delay  en=off  latency=3  dbl_ovrd=off  reg_retiming=off  block_type=delay
      settings: block_version=11.4
  delay_we : xbsIndex_r4/Delay  en=off  latency=0  dbl_ovrd=off  reg_retiming=off  block_type=delay
      settings: block_version=11.4
  map1 : xbsIndex_r4/ROM  depth=128  initVector=[0 64 32 96 16 80 48 112 8 72 40 104 24 88 56 120 4 68 36 100 20 84 52 116 12 76 44 108 28 92 60 124 2 66 34 98 18 82 50 114 10 74 42 106 26 90 58 122 6 70 38 102 22 86 54 118 14 78 46 110 30 94 62 126 1 65 33 97 17 81 49 113 9 73 41 105 25 89 57 121 5 69 37 101 21 85 53 117 13 77 45 109 29 93 61 125 3 67 35 99 19 83 51 115 11 75 43 107 27 91 59 123 7 71 39 103 23 87 55 119 15 79 47 111 31 95 63 127]  distributed_mem=Distributed memory  rst=off  init_reg=0  en=off  latency=0  arith_type=Unsigned  n_bits=7  bin_pt=0  dbl_ovrd=off  optimize=Area  use_rpm=on  block_type=sprom
      settings: block_version=11.4
  post_sync_delay : xbsIndex_r4/Delay  en=off  latency=3  dbl_ovrd=off  reg_retiming=off  block_type=delay
      settings: block_version=11.4
  pre_sync_delay : xbsIndex_r4/Delay  en=off  latency=0  dbl_ovrd=off  reg_retiming=off  block_type=delay
      settings: block_version=11.4
  sync_delay_en : Subsystem
  sync_out : Outport
  valid : Outport  Port=2
  dout0 : Outport  Port=3
  wires:
  sync/1 -> Counter/1, pre_sync_delay/1
  en/1 -> Counter/2, delay_we/1, sync_delay_en/2(en)
  delay_we/1 -> bram0/3, delay_valid/1
  Counter/1 -> Slice2/1, Slice1/1
  Slice2/1 -> map1/1, delay_d0/1
  delay_map1/1 -> Mux/3
  map1/1 -> delay_map1/1
  bram0/1 -> dout0/1
  delay_din0/1 -> bram0/2
  Mux/1 -> bram0/1
  din0/1 -> delay_din0/1
  delay_d0/1 -> Mux/2
  delay_sel/1 -> Mux/1
  Slice1/1 -> delay_sel/1
  delay_valid/1 -> valid/1
  post_sync_delay/1 -> sync_out/1
  sync_delay_en/1(Out) -> post_sync_delay/1
  pre_sync_delay/1 -> sync_delay_en/1(In)

== system xblocks_library_ffts_internal/bi_real_unscr_4x/reorder_odd ==
  sync : Inport
  en : Inport  Port=2
  din0 : Inport  Port=3
  Counter : xbsIndex_r4/Counter  cnt_type=Count Limited  cnt_to=255  operation=Up  start_count=0  cnt_by_val=1  arith_type=Unsigned  n_bits=8  bin_pt=0  load_pin=off  rst=on  en=on  explicit_period=on  period=1  dbl_ovrd=off  use_behavioral_HDL=off  implementation=Fabric  block_type=counter
      settings: block_version=11.4
  Mux : xbsIndex_r4/Mux  inputs=2  en=off  latency=1  precision=Full  arith_type=Unsigned  n_bits=16  bin_pt=14  quantization=Truncate  overflow=Wrap  dbl_ovrd=off  block_type=mux
      settings: block_version=11.4
  Slice1 : xbsIndex_r4/Slice  nbits=1  boolean_output=off  mode=Upper Bit Location + Width  bit1=0  base1=MSB of Input  bit0=0  base0=LSB of Input  dbl_ovrd=off  block_type=slice
  Slice2 : xbsIndex_r4/Slice  nbits=7  boolean_output=off  mode=Lower Bit Location + Width  bit1=0  base1=MSB of Input  bit0=0  base0=LSB of Input  dbl_ovrd=off  block_type=slice
  bram0 : xbsIndex_r4/Single Port RAM  depth=128  initVector=sin(pi*(0:15)/16)  distributed_mem=Block RAM  write_mode=Read Before Write  rst=off  init_reg=0  en=off  latency=2  dbl_ovrd=off  optimize=Area  use_rpm=on  block_type=spram
  delay_d0 : xbsIndex_r4/Delay  en=off  latency=0  dbl_ovrd=off  reg_retiming=off  block_type=delay
      settings: block_version=11.4
  delay_din0 : xbsIndex_r4/Delay  en=off  latency=1  dbl_ovrd=off  reg_retiming=off  block_type=delay
      settings: block_version=11.4
  delay_map1 : xbsIndex_r4/Delay  en=off  latency=0  dbl_ovrd=off  reg_retiming=off  block_type=delay
      settings: block_version=11.4
  delay_sel : xbsIndex_r4/Delay  en=off  latency=0  dbl_ovrd=off  reg_retiming=off  block_type=delay
      settings: block_version=11.4
  delay_valid : xbsIndex_r4/Delay  en=off  latency=3  dbl_ovrd=off  reg_retiming=off  block_type=delay
      settings: block_version=11.4
  delay_we : xbsIndex_r4/Delay  en=off  latency=0  dbl_ovrd=off  reg_retiming=off  block_type=delay
      settings: block_version=11.4
  map1 : xbsIndex_r4/ROM  depth=128  initVector=[127 63 95 31 111 47 79 15 119 55 87 23 103 39 71 7 123 59 91 27 107 43 75 11 115 51 83 19 99 35 67 3 125 61 93 29 109 45 77 13 117 53 85 21 101 37 69 5 121 57 89 25 105 41 73 9 113 49 81 17 97 33 65 1 126 62 94 30 110 46 78 14 118 54 86 22 102 38 70 6 122 58 90 26 106 42 74 10 114 50 82 18 98 34 66 2 124 60 92 28 108 44 76 12 116 52 84 20 100 36 68 4 120 56 88 24 104 40 72 8 112 48 80 16 96 32 64 0]  distributed_mem=Distributed memory  rst=off  init_reg=0  en=off  latency=0  arith_type=Unsigned  n_bits=7  bin_pt=0  dbl_ovrd=off  optimize=Area  use_rpm=on  block_type=sprom
      settings: block_version=11.4
  post_sync_delay : xbsIndex_r4/Delay  en=off  latency=3  dbl_ovrd=off  reg_retiming=off  block_type=delay
      settings: block_version=11.4
  pre_sync_delay : xbsIndex_r4/Delay  en=off  latency=0  dbl_ovrd=off  reg_retiming=off  block_type=delay
      settings: block_version=11.4
  sync_delay_en : Subsystem
  sync_out : Outport
  valid : Outport  Port=2
  dout0 : Outport  Port=3
  wires:
  sync/1 -> Counter/1, pre_sync_delay/1
  en/1 -> Counter/2, delay_we/1, sync_delay_en/2(en)
  delay_we/1 -> bram0/3, delay_valid/1
  Counter/1 -> Slice2/1, Slice1/1
  Slice2/1 -> map1/1, delay_d0/1
  delay_map1/1 -> Mux/3
  map1/1 -> delay_map1/1
  bram0/1 -> dout0/1
  delay_din0/1 -> bram0/2
  Mux/1 -> bram0/1
  din0/1 -> delay_din0/1
  delay_d0/1 -> Mux/2
  delay_sel/1 -> Mux/1
  Slice1/1 -> delay_sel/1
  delay_valid/1 -> valid/1
  post_sync_delay/1 -> sync_out/1
  sync_delay_en/1(Out) -> post_sync_delay/1
  pre_sync_delay/1 -> sync_delay_en/1(In)

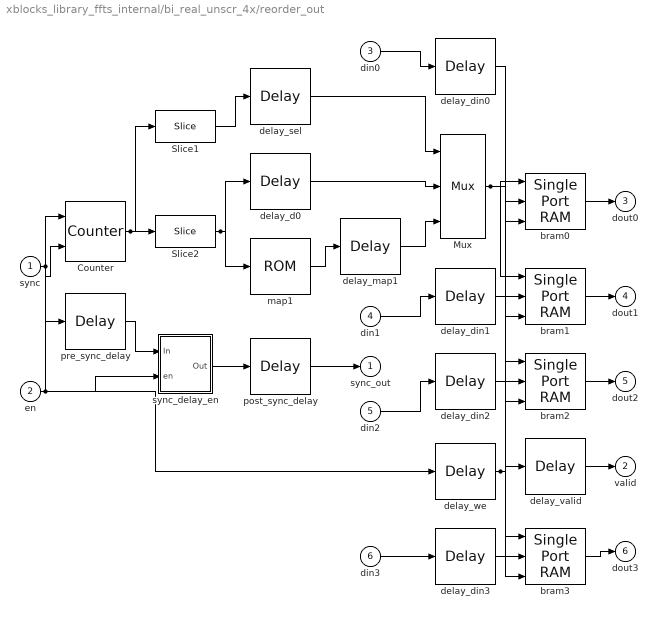
== system xblocks_library_ffts_internal/bi_real_unscr_4x/reorder_out ==
  sync : Inport
  en : Inport  Port=2
  din0 : Inport  Port=3
  din1 : Inport  Port=4
  din2 : Inport  Port=5
  din3 : Inport  Port=6
  Counter : xbsIndex_r4/Counter  cnt_type=Count Limited  cnt_to=255  operation=Up  start_count=0  cnt_by_val=1  arith_type=Unsigned  n_bits=8  bin_pt=0  load_pin=off  rst=on  en=on  explicit_period=on  period=1  dbl_ovrd=off  use_behavioral_HDL=off  implementation=Fabric  block_type=counter
      settings: block_version=11.4
  Mux : xbsIndex_r4/Mux  inputs=2  en=off  latency=1  precision=Full  arith_type=Unsigned  n_bits=16  bin_pt=14  quantization=Truncate  overflow=Wrap  dbl_ovrd=off  block_type=mux
      settings: block_version=11.4
  Slice1 : xbsIndex_r4/Slice  nbits=1  boolean_output=off  mode=Upper Bit Location + Width  bit1=0  base1=MSB of Input  bit0=0  base0=LSB of Input  dbl_ovrd=off  block_type=slice
  Slice2 : xbsIndex_r4/Slice  nbits=7  boolean_output=off  mode=Lower Bit Location + Width  bit1=0  base1=MSB of Input  bit0=0  base0=LSB of Input  dbl_ovrd=off  block_type=slice
  bram{0..3} (4 alike) : xbsIndex_r4/Single Port RAM  depth=128  initVector=sin(pi*(0:15)/16)  distributed_mem=Block RAM  write_mode=Read Before Write  rst=off  init_reg=0  en=off  latency=2  dbl_ovrd=off  optimize=Area  use_rpm=on  block_type=spram
  delay_d0 : xbsIndex_r4/Delay  en=off  latency=0  dbl_ovrd=off  reg_retiming=off  block_type=delay
      settings: block_version=11.4
  delay_din{0..3} (4 alike) : xbsIndex_r4/Delay  en=off  latency=1  dbl_ovrd=off  reg_retiming=off  block_type=delay
      settings: block_version=11.4
  delay_map1 : xbsIndex_r4/Delay  en=off  latency=0  dbl_ovrd=off  reg_retiming=off  block_type=delay
      settings: block_version=11.4
  delay_sel : xbsIndex_r4/Delay  en=off  latency=0  dbl_ovrd=off  reg_retiming=off  block_type=delay
      settings: block_version=11.4
  delay_valid : xbsIndex_r4/Delay  en=off  latency=3  dbl_ovrd=off  reg_retiming=off  block_type=delay
      settings: block_version=11.4
  delay_we : xbsIndex_r4/Delay  en=off  latency=0  dbl_ovrd=off  reg_retiming=off  block_type=delay
      settings: block_version=11.4
  map1 : xbsIndex_r4/ROM  depth=128  initVector=[127 126 125 124 123 122 121 120 119 118 117 116 115 114 113 112 111 110 109 108 107 106 105 104 103 102 101 100 99 98 97 96 95 94 93 92 91 90 89 88 87 86 85 84 83 82 81 80 79 78 77 76 75 74 73 72 71 70 69 68 67 66 65 64 63 62 61 60 59 58 57 56 55 54 53 52 51 50 49 48 47 46 45 44 43 42 41 40 39 38 37 36 35 34 33 32 31 30 29 28 27 26 25 24 23 22 21 20 19 18 17 16 15 14 13 12 11 10 9 8 7 6 5 4 3 2 1 0]  distributed_mem=Distributed memory  rst=off  init_reg=0  en=off  latency=0  arith_type=Unsigned  n_bits=7  bin_pt=0  dbl_ovrd=off  optimize=Area  use_rpm=on  block_type=sprom
      settings: block_version=11.4
  post_sync_delay : xbsIndex_r4/Delay  en=off  latency=3  dbl_ovrd=off  reg_retiming=off  block_type=delay
      settings: block_version=11.4
  pre_sync_delay : xbsIndex_r4/Delay  en=off  latency=0  dbl_ovrd=off  reg_retiming=off  block_type=delay
      settings: block_version=11.4
  sync_delay_en : Subsystem
  sync_out : Outport
  valid : Outport  Port=2
  dout0 : Outport  Port=3
  dout1 : Outport  Port=4
  dout2 : Outport  Port=5
  dout3 : Outport  Port=6
  wires:
  sync/1 -> Counter/1, pre_sync_delay/1
  en/1 -> Counter/2, delay_we/1, sync_delay_en/2(en)
  delay_we/1 -> bram3/3, bram2/3, bram1/3, bram0/3, delay_valid/1
  Counter/1 -> Slice2/1, Slice1/1
  Slice2/1 -> map1/1, delay_d0/1
  Mux/1 -> bram3/1, bram2/1, bram1/1, bram0/1
  delay_map1/1 -> Mux/3
  map1/1 -> delay_map1/1
  bram3/1 -> dout3/1
  delay_din3/1 -> bram3/2
  din3/1 -> delay_din3/1
  bram2/1 -> dout2/1
  delay_din2/1 -> bram2/2
  din2/1 -> delay_din2/1
  bram1/1 -> dout1/1
  delay_din1/1 -> bram1/2
  din1/1 -> delay_din1/1
  bram0/1 -> dout0/1
  delay_din0/1 -> bram0/2
  din0/1 -> delay_din0/1
  delay_d0/1 -> Mux/2
  delay_sel/1 -> Mux/1
  Slice1/1 -> delay_sel/1
  delay_valid/1 -> valid/1
  post_sync_delay/1 -> sync_out/1
  sync_delay_en/1(Out) -> post_sync_delay/1
  pre_sync_delay/1 -> sync_delay_en/1(In)

== system xblocks_library_ffts_internal/bi_real_unscr_4x/sync_delay_ctr ==
  In : Inport
      settings: AttributesFormatString=18_17 r/i
  Constant : xbsIndex_r4/Constant  arith_type=Unsigned  const=1  n_bits=8  bin_pt=0  explicit_period=on  period=1  equ=P=C  opselect=C  inp2=PCIN>>17  opr=+  inp1=P  carry=CIN  dbl_ovrd=off  block_type=constant
      settings: block_version=11.4
  Constant1 : xbsIndex_r4/Constant  arith_type=Unsigned  const=0  n_bits=8  bin_pt=0  explicit_period=on  period=1  equ=P=C  opselect=C  inp2=PCIN>>17  opr=+  inp1=P  carry=CIN  dbl_ovrd=off  block_type=constant
      settings: block_version=11.4
  Constant2 : xbsIndex_r4/Constant  arith_type=Unsigned  const=131  n_bits=8  bin_pt=0  explicit_period=on  period=1  equ=P=C  opselect=C  inp2=PCIN>>17  opr=+  inp1=P  carry=CIN  dbl_ovrd=off  block_type=constant
      settings: block_version=11.4
  Constant3 : xbsIndex_r4/Constant  arith_type=Unsigned  const=1  n_bits=1  bin_pt=0  explicit_period=on  period=1  equ=P=C  opselect=C  inp2=PCIN>>17  opr=+  inp1=P  carry=CIN  dbl_ovrd=off  block_type=constant
      settings: block_version=11.4
  Counter : xbsIndex_r4/Counter  cnt_type=Free Running  cnt_to=Inf  operation=Down  start_count=0  cnt_by_val=1  arith_type=Unsigned  n_bits=8  bin_pt=0  load_pin=on  rst=off  en=on  explicit_period=on  period=1  dbl_ovrd=off  use_behavioral_HDL=off  implementation=Fabric  use_rpm=on  block_type=counter
      settings: block_version=11.4
  Logical : xbsIndex_r4/Logical  logical_function=OR  inputs=2  en=off  latency=0  precision=Full  arith_type=Unsigned  n_bits=8  bin_pt=2  align_bp=on  dbl_ovrd=off  block_type=logical
      settings: block_version=11.4
  Mux : xbsIndex_r4/Mux  inputs=2  en=off  latency=0  precision=Full  arith_type="Signed  (2's comp)"  n_bits=8  bin_pt=2  quantization=Truncate  overflow=Wrap  dbl_ovrd=off  block_type=mux
      settings: block_version=11.4
  Relational : xbsIndex_r4/Relational  mode=a=b  en=off  latency=0  dbl_ovrd=off  block_type=relational
  Relational1 : xbsIndex_r4/Relational  mode=a!=b  en=off  latency=0  dbl_ovrd=off  block_type=relational
  Out : Outport
  wires:
  In/1 -> Mux/2, Logical/1, Counter/1
  Counter/1 -> Relational1/1, Relational/2
  Relational1/1 -> Logical/2
  Constant1/1 -> Relational1/2
  Relational/1 -> Mux/3
  Constant/1 -> Relational/1
  Mux/1 -> Out/1
  Constant3/1 -> Mux/1
  Logical/1 -> Counter/3
  Constant2/1 -> Counter/2

== system xblocks_library_ffts_internal/hilbert/c_to_ri ==
  c : Inport
  force_im : xbsIndex_r4/Reinterpret  force_arith_type=on  arith_type="Signed  (2's comp)"  force_bin_pt=on  bin_pt=15  block_type=reinterpret
      settings: infoedit="Changes signal type without altering the binary representation.   You can changed the signal between signed and unsigned, and relocate the binary point.<br><br>Hardware notes: In hardware this block costs nothing.<br><br>Example:  Suppose the input is 6 bits wide, signed, with 2 fractional bits, and the output is forced to unsigned with 0 fractional bits.  Then an input of -2.0 (1110.00 in binary 2's complement) becomes an output of 56 (111000 in binary)."
  force_re : xbsIndex_r4/Reinterpret  force_arith_type=on  arith_type="Signed  (2's comp)"  force_bin_pt=on  bin_pt=15  block_type=reinterpret
      settings: infoedit="Changes signal type without altering the binary representation.   You can changed the signal between signed and unsigned, and relocate the binary point.<br><br>Hardware notes: In hardware this block costs nothing.<br><br>Example:  Suppose the input is 6 bits wide, signed, with 2 fractional bits, and the output is forced to unsigned with 0 fractional bits.  Then an input of -2.0 (1110.00 in binary 2's complement) becomes an output of 56 (111000 in binary)."
  slice_im : xbsIndex_r4/Slice  nbits=16  boolean_output=off  mode=Lower Bit Location + Width  bit1=0  base1=MSB of Input  bit0=0  base0=LSB of Input  dbl_ovrd=off  block_type=slice
  slice_re : xbsIndex_r4/Slice  nbits=16  boolean_output=off  mode=Upper Bit Location + Width  bit1=0  base1=MSB of Input  bit0=0  base0=LSB of Input  dbl_ovrd=off  block_type=slice
  re : Outport
  im : Outport  Port=2
  wires:
  c/1 -> slice_re/1, slice_im/1
  slice_re/1 -> force_re/1
  slice_im/1 -> force_im/1
  force_re/1 -> re/1
  force_im/1 -> im/1
